simulink model "trms_paper_ind_withfuncblock_integrator_varying_plant"  (R2024a)
settings: Solver=VariableStepAuto  StartTime=0.0  StopTime=1100  RelTol=1e-9
values from neighbouring files (symbols this model uses):
  Aam = [0 1 0 0 0 0 ... (first row only)    [trms_paper.m]
  alpha = 10    [trms_paper.m]
  Bam = [zeros(4,2) ... (first row only)    [trms_paper.m]
  gama = 500    [trms_paper.m]
  lamda = 2    [trms_paper.m]
settings Model: Creator=Unnati  LastModifiedBy=Unnati

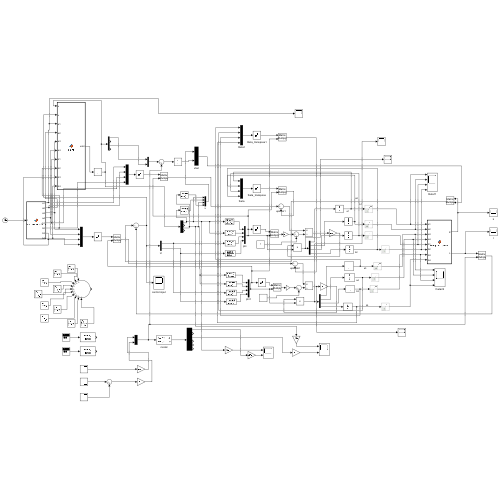
[thumbnail: Simulink's stored preview of the top-level diagram]
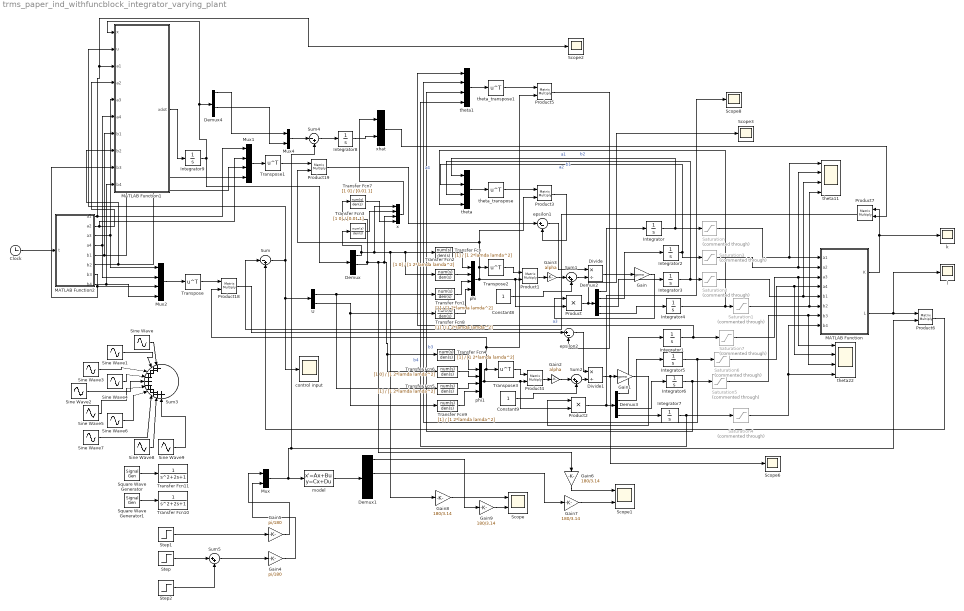
== system trms_paper_ind_withfuncblock_integrator_varying_plant ==
  Clock : Clock
  Constant8 : Constant
  Constant9 : Constant
  Demux{,2..4} (4 alike) : Demux
  Demux1 : Demux  Outputs=6
  Divide : Product  Inputs=*/
  Divide1 : Product  Inputs=*/
  Gain : Gain  Gain=gama
  Gain1 : Gain  Gain=gama
  Gain2 : Gain  Gain=alpha
  Gain3 : Gain  Gain=alpha
  Gain4 : Gain  Gain=pi/180
  Gain5 : Gain  Gain=pi/180
  Gain{6..9} (4 alike) : Gain  Gain=180/3.14
  Integrator : Integrator  InitialCondition=1.5
  Integrator1 : Integrator  InitialCondition=0.2
  Integrator2 : Integrator  InitialCondition=0.25
  Integrator3 : Integrator  InitialCondition=0.04
  Integrator4 : Integrator  InitialCondition=0.08
  Integrator5 : Integrator  InitialCondition=0.8
  Integrator6 : Integrator  InitialCondition=-0.1
  Integrator7 : Integrator  InitialCondition=0.08
  Integrator8 : Integrator
  Integrator9 : Integrator
  MATLAB Function : MATLAB Function  TreatAsAtomicUnit=on
  MATLAB Function1 : MATLAB Function  TreatAsAtomicUnit=on
  MATLAB Function2 : MATLAB Function  TreatAsAtomicUnit=on
  Mux : Mux  Inputs=2
  Mux1 : Mux
  Mux2 : Mux
  Mux4 : Mux  Inputs=2
  Product : Product
  Product{1,3..7,18..19} (8 alike) : Product  Multiplication=Matrix(*)
  Product2 : Product
  Saturation : Saturate  Commented=through  UpperLimit=3  LowerLimit=0.5
  Saturation1 : Saturate  Commented=through  UpperLimit=0.2  LowerLimit=0.1
  Saturation2 : Saturate  Commented=through  UpperLimit=0.1  LowerLimit=0.01
  Saturation3 : Saturate  Commented=through  UpperLimit=2  LowerLimit=0
  Saturation4 : Saturate  Commented=through  UpperLimit=0.2  LowerLimit=0.01
  Saturation5 : Saturate  Commented=through  UpperLimit=0.01  LowerLimit=-0.2
  Saturation6 : Saturate  Commented=through  UpperLimit=2  LowerLimit=0
  Saturation7 : Saturate  Commented=through  UpperLimit=1  LowerLimit=-1
  Scope : Scope  NumInputPorts=2
  Scope1 : Scope  NumInputPorts=2
  Scope{2..3,6,8} (4 alike) : Scope
  Sine Wave : Sin  SampleTime=0
  Sine Wave1 : Sin  Amplitude=2  Frequency=2  SampleTime=0
  Sine Wave2 : Sin  Amplitude=5  Frequency=5  SampleTime=0
  Sine Wave3 : Sin  Amplitude=3  Frequency=3  SampleTime=0
  Sine Wave4 : Sin  Amplitude=4  Frequency=4  SampleTime=0
  Sine Wave5 : Sin  Amplitude=6  Frequency=6  SampleTime=0
  Sine Wave6 : Sin  Amplitude=7  Frequency=7  SampleTime=0
  Sine Wave7 : Sin  Amplitude=8  Frequency=8  SampleTime=0
  Sine Wave8 : Sin  Amplitude=9  Frequency=9  SampleTime=0
  Sine Wave9 : Sin  Amplitude=10  Frequency=10  SampleTime=0
  Square Wave Generator : SignalGenerator  WaveForm=square  Frequency=0.05
  Square Wave Generator1 : SignalGenerator  WaveForm=square  Frequency=0.05
  Step : Step  Time=600  Before=10  After=0  SampleTime=0
  Step1 : Step  Time=0  After=10  SampleTime=0
  Step2 : Step  Time=1000  After=10  SampleTime=0
  Sum : Sum  Inputs=|-+
  Sum1 : Sum  Inputs=|++
  Sum2 : Sum  Inputs=|++
  Sum3 : Sum  Inputs=|++++++++++
  Sum4 : Sum  Inputs=|-+
  Sum5 : Sum  Inputs=|++
  Transfer Fcn{,1,4..5,8..9} (6 alike) : TransferFcn  Denominator=[1 2*lamda lamda^2]
  Transfer Fcn10 : TransferFcn
  Transfer Fcn11 : TransferFcn
  Transfer Fcn2 : TransferFcn  Numerator=[1 0]  Denominator=[1 2*lamda lamda^2]
  Transfer Fcn3 : TransferFcn  Numerator=[1 0]  Denominator=[0.01 1]
  Transfer Fcn6 : TransferFcn  Numerator=[1 0]  Denominator=[1 2*lamda lamda^2]
  Transfer Fcn7 : TransferFcn  Numerator=[1 0]  Denominator=[0.01 1]
  Transpose{,1..3} (4 alike) : Math  Operator=transpose
  U : Demux  Outputs=2
  control input : Scope
  epsilon1 : Sum  Inputs=|+-
  epsilon2 : Sum  Inputs=|+-
  k : Scope
  l : Scope
  model : StateSpace  A=Aam  B=Bam  C=eye(6)  D=zeros(6,2)  InitialCondition=0
  phi : Mux
  phi1 : Mux
  theta : Mux
  theta1 : Mux
  theta11 : Scope  NumInputPorts=4
  theta22 : Scope  NumInputPorts=4
  theta_transpose : Math  Operator=transpose
  theta_transpose1 : Math  Operator=transpose
  x : Mux
  xhat : Mux  Inputs=2
  wires:
  Gain7/1 -> Scope1/2
  Demux2/1 -> Integrator/1
  Demux/1 -> Transfer Fcn3/1, x/1, Gain8/1, Transfer Fcn2/1, Transfer Fcn/1
  Square Wave Generator1/1 -> Transfer Fcn10/1
  Gain8/1 -> Scope/1
  Gain/1 -> Product/1
  Sine Wave9/1 -> Sum3/10
  Sine Wave8/1 -> Sum3/9
  Demux3/4 -> Integrator7/1
  Saturation5/1 -> theta22/3, MATLAB Function/7(b3)
  theta/1 -> theta_transpose/1
  Gain9/1 -> Scope/2
  Integrator2/1 -> theta/2, Saturation3/1  "a2"
  Demux/3 -> Transfer Fcn7/1, Gain6/1, x/3, Transfer Fcn6/1, Transfer Fcn4/1
  Sine Wave7/1 -> Sum3/8
  Gain3/1 -> Sum1/1
  Sine Wave3/1 -> Sum3/3
  Demux1/3 -> Gain7/1
  Saturation/1 -> theta11/1, MATLAB Function/1(a1)
  MATLAB Function/1(K) -> k/1, Product7/1
  Sine Wave6/1 -> Sum3/7
  xhat/1 -> Product7/2
  Demux3/1 -> Integrator1/1
  Saturation7/1 -> theta22/1, MATLAB Function/3(a3)
  Sum1/1 -> Divide/2
  Product6/1 -> Sum/2
  Demux3/2 -> Integrator5/1
  Transpose3/1 -> Product4/1
  Product3/1 -> epsilon1/2
  Constant9/1 -> Sum2/2
  epsilon2/1 -> Divide1/1
  Mux4/1 -> Sum4/1
  Transfer Fcn8/1 -> phi/4
  U/1 -> Transfer Fcn5/1, Transfer Fcn1/1
  Sine Wave1/1 -> Sum3/2
  theta_transpose/1 -> Product3/1
  Transpose1/1 -> Product19/1
  Sine Wave2/1 -> Sum3/5
  Sum4/1 -> Integrator8/1
  Integrator8/1 -> xhat/2
  Demux1/1 -> Gain9/1
  Product2/1 -> Scope8/1, Demux3/1
  Integrator5/1 -> theta1/2, Saturation6/1  "a4"
  Gain6/1 -> Scope1/1
  Integrator6/1 -> theta1/3, Saturation5/1  "b3"
  Divide/1 -> Gain/1
  Transfer Fcn2/1 -> phi/2
  Saturation1/1 -> theta11/4, MATLAB Function/6(b2)
  Constant8/1 -> Sum1/2
  Integrator/1 -> theta/1, Saturation/1  "a1"
  Transfer Fcn9/1 -> phi1/4
  Product18/1 -> epsilon2/1
  Integrator7/1 -> Saturation4/1, theta1/4  "b4"
  Gain2/1 -> Sum2/1
  Square Wave Generator/1 -> Transfer Fcn11/1
  Transfer Fcn3/1 -> x/2
  epsilon1/1 -> Divide/1
  Transpose2/1 -> Product1/1
  U/2 -> Transfer Fcn9/1, Transfer Fcn8/1
  Product/1 -> Scope3/1, Demux2/1
  Transfer Fcn/1 -> phi/1
  model/1 -> Demux1/1
  Product4/1 -> Gain2/1
  Transfer Fcn1/1 -> phi/3
  MATLAB Function/2(L) -> l/1, Product6/1
  Integrator1/1 -> theta1/1, Saturation7/1  "a3"
  Saturation6/1 -> theta22/2, MATLAB Function/4(a4)
  Integrator3/1 -> theta/3, Saturation2/1  "b1"
  Integrator4/1 -> theta/4, Saturation1/1  "b2"
  Transfer Fcn4/1 -> phi1/1
  Saturation3/1 -> theta11/2, MATLAB Function/2(a2)
  Mux2/1 -> Transpose/1
  Product7/1 -> Sum/1
  Saturation4/1 -> MATLAB Function/8(b4), theta22/4
  Divide1/1 -> Scope6/1, Gain1/1
  Demux2/3 -> Integrator3/1
  Mux1/1 -> Transpose1/1
  Gain5/1 -> Mux/1
  Sum/1 -> control input/1, U/1, MATLAB Function1/2(u)
  Sine Wave5/1 -> Sum3/6
  theta_transpose1/1 -> Product5/1
  Product5/1 -> epsilon2/2
  Sum2/1 -> Divide1/2
  Sine Wave4/1 -> Sum3/4
  Product19/1 -> epsilon1/1
  Sine Wave/1 -> Sum3/1
  phi1/1 -> Product18/2, Product5/2, Transpose3/1, Product2/2, Product4/2
  Transfer Fcn7/1 -> x/4
  Demux3/3 -> Integrator6/1
  theta1/1 -> theta_transpose1/1
  Demux2/4 -> Integrator4/1
  Transpose/1 -> Product18/1
  phi/1 -> Product19/2, Product3/2, Transpose2/1, Product/2, Product1/2
  Demux2/2 -> Integrator2/1
  Mux/1 -> model/1, Product6/2, Sum4/2
  Product1/1 -> Gain3/1
  Transfer Fcn5/1 -> phi1/3
  Gain1/1 -> Product2/1
  Transfer Fcn6/1 -> phi1/2
  Saturation2/1 -> theta11/3, MATLAB Function/5(b1)
  Clock/1 -> MATLAB Function2/1("t ")
  MATLAB Function1/1(xdot) -> Integrator9/1
  Demux4/1 -> Mux4/1
  Demux4/3 -> Mux4/2
  Integrator9/1 -> MATLAB Function1/1(x), Demux4/1, Demux/1
  MATLAB Function2/1(a1) -> Mux1/1, Scope2/1, MATLAB Function1/3(a1)
  MATLAB Function2/2(a2) -> MATLAB Function1/4(a2), Mux1/2
  MATLAB Function2/5(b1) -> MATLAB Function1/7(b1), Mux1/3
  MATLAB Function2/6(b2) -> MATLAB Function1/8(b2), Mux1/4
  MATLAB Function2/3(a3) -> Mux2/1, MATLAB Function1/5(a3)
  MATLAB Function2/4(a4) -> Mux2/2, MATLAB Function1/6(a4)
  MATLAB Function2/7(b3) -> MATLAB Function1/9(b3), Mux2/3
  MATLAB Function2/8(b4) -> MATLAB Function1/10(b4), Mux2/4
  x/1 -> xhat/1
  Gain4/1 -> Mux/2
  Step/1 -> Sum5/1
  Step2/1 -> Sum5/2
  Sum5/1 -> Gain4/1
  Step1/1 -> Gain5/1

== matlab function trms_paper_ind_withfuncblock_integrator_varying_plant/MATLAB Function1 ==
  data: x input; u input; xdot output; a1 input; a2 input; a3 input; a4 input; b1 input; b2 input; b3 input; b4 input
function xdot = plant(x,u,a1,a2,a3,a4,b1,b2,b3,b4)

xdot = zeros(4,1);

xdot(1) = x(2);

xdot(2) = -a1*x(1) - a2*x(2) ...
          + b1*u(1) + b2*u(2);

xdot(3) = x(4);

xdot(4) = -a3*x(3) - a4*x(4) ...
          + b3*u(1) + b4*u(2);

end

== matlab function trms_paper_ind_withfuncblock_integrator_varying_plant/MATLAB Function ==
  settings: updateMethod=DISCRETE
  data: a1 input; K output size=[2 6]; a2 input; a3 input; a4 input; b1 input; b2 input; b3 input; b4 input; L output size=[2 2]
function [K,L] = compute_gains(a1,a2,a3,a4,b1,b2,b3,b4)

% a1= 1.71;
% a2= 0.32;
% b1= 0.05;
% b2= 0.095;
% a3= 0;
% a4= 1;
% b3= -0.12;
% b4= 0.1;

K = zeros(2,6);
L = zeros(2,2);

Ahat = [0 1 0 0;
       -a1 -a2 0 0;
        0 0 0 1;
        0 0 -a3 -a4];

Bhat = [0 0;
        b1 b2;
        0 0;
        b3 b4];

C = [1 0 0 0;
     0 0 1 0];

% Am = [0 1 0 0;
%      -4 -2 0 0;
%       0 0 0 1;
%       0 0 -4 -2];
% 
% Bm = [0 0;
%       4 0;
%       0 0;
%       0 4];

Aaug = [Ahat zeros(4,2);
        -C  zeros(2,2)];

Baug = [Bhat;
        zeros(2,2)];


Aam = [0 1 0 0 0 0;
      -8 -4 0 0 8 0;
       0 0 0 1 0 0;
       0 0 -8 -4 0 8;
       -1 0 0 0 0 0;
       0 0 -1 0 0 0];

Bam = [zeros(4,2);
       eye(2)];


Delta = Aaug - Aam;

Binv = (inv(Baug'*Baug))*(Baug)';

% K = Binv*Delta;
% L = Binv*Bam;
K = pinv(Baug)*Delta;
L = pinv(Baug)*Bam;

== matlab function trms_paper_ind_withfuncblock_integrator_varying_plant/MATLAB Function2 ==
  data: t input; a1 output; a2 output; a3 output; a4 output; b1 output; b2 output; b3 output; b4 output
function [a1,a2,a3,a4,b1,b2,b3,b4] = true_parameters(t)

% Nominal true parameters
a1_nom = 1.71;
a2_nom = 0.32;
a3_nom = 0;
a4_nom = 1;

b1_nom = 0.05;
b2_nom = 0.095;
b3_nom = -0.12;
b4_nom = 0.1;

if t < 400

    a1 = a1_nom;
    a2 = a2_nom;
    a3 = a3_nom;
    a4 = a4_nom;

    b1 = b1_nom;
    b2 = b2_nom;
    b3 = b3_nom;
    b4 = b4_nom;

else

    a1 = 1*a1_nom;
    a2 = 1.2*a2_nom;
    a3 = 1.5*a3_nom;
    a4 = -0.8*a4_nom;

    b1 = 1*b1_nom;
    b2 = 1.2*b2_nom;
    b3 = 1.9*b3_nom;
    b4 = 1.1*b4_nom;

end
